simulink model "Grundregler"  (R2018b)
settings: Solver=VariableStepAuto  StartTime=0.0  StopTime=10.0  RelTol=1e-3
settings Model: Creator=F58925B  LastModifiedBy=F58925B

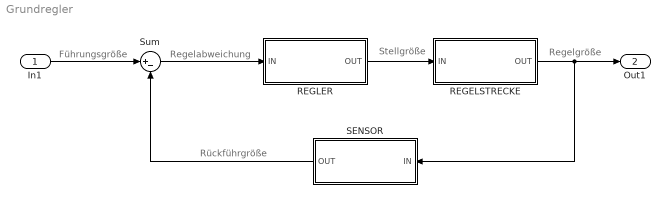
== system Grundregler ==
  note: Regelgröße
  note: Stellgröße
  note: Regelabweichung
  note: Führungsgröße
  note: Rückführgröße
  In1 : Inport
  REGELSTRECKE : Subsystem
  REGLER : Subsystem
  SENSOR : Subsystem
  Sum : Sum  Inputs=|+-
  Out1 : Outport  Port=2
  wires:
  REGELSTRECKE/1(OUT) -> Out1/1, SENSOR/1(IN)
  REGLER/1(OUT) -> REGELSTRECKE/1(IN)
  Sum/1 -> REGLER/1(IN)
  In1/1 -> Sum/1
  SENSOR/1(OUT) -> Sum/2

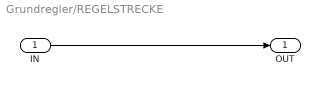
== system Grundregler/REGELSTRECKE ==
  IN : Inport
  OUT : Outport
  wires:
  IN/1 -> OUT/1

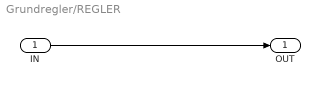
== system Grundregler/REGLER ==
  IN : Inport
  OUT : Outport
  wires:
  IN/1 -> OUT/1

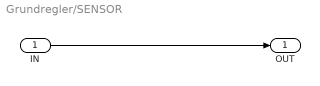
== system Grundregler/SENSOR ==
  IN : Inport
  OUT : Outport
  wires:
  IN/1 -> OUT/1
